simulink model "Cruise_Control_Plant"  (R2020b)
settings: Solver=VariableStepAuto  StartTime=0.0  StopTime=10  RelTol=1e-3
undefined symbols (not defined in the file or in its folder): b, m
settings Model: DataDictionary=Problem3_data.sldd  Creator=ASUS  LastModifiedBy=ASUS
settings DataIOCC: SaveOutput=off  SaveTime=off

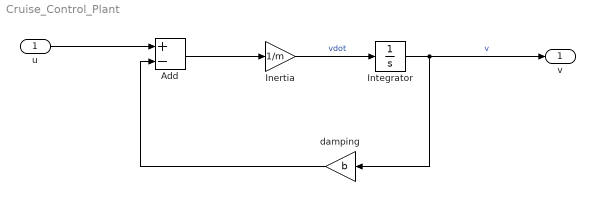
== system Cruise_Control_Plant ==
  u : Inport  OutDataTypeStr=double  PortDimensions=1  SampleTime=0
  Add : Sum  Inputs=+-
  Inertia : Gain  Gain=1/m
  Integrator : Integrator
  damping : Gain  Gain=b
  v : Outport  OutDataTypeStr=double  PortDimensions=1  SampleTime=0
  wires:
  Add/1 -> Inertia/1
  Integrator/1 -> damping/1, v/1  "v"
  u/1 -> Add/1
  damping/1 -> Add/2
  Inertia/1 -> Integrator/1  "vdot"
